simulink model "SEMINAR_DFIG_GSC_Controller"  (R2014a)
settings: Solver=ode45  StartTime=0.0  StopTime=10.0  RelTol=1e-3
libraries: powerlib_meascontrol x12, simulink x6
settings Model: Creator=user  LastModifiedBy=ninad gaikawad

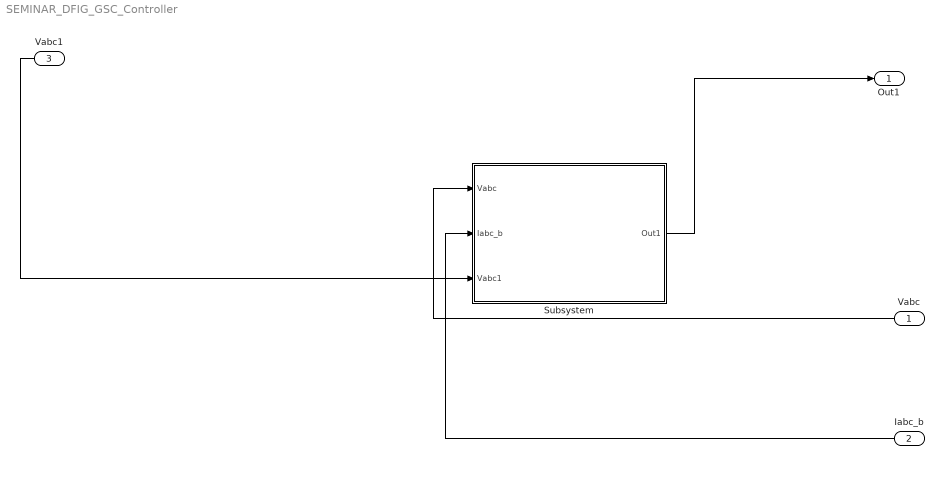
== system SEMINAR_DFIG_GSC_Controller ==
  Vabc : Inport
  Iabc_b : Inport  Port=2
  Vabc1 : Inport  Port=3
  Subsystem : Subsystem
  Out1 : Outport
  wires:
  Vabc/1 -> Subsystem/1(Vabc)
  Iabc_b/1 -> Subsystem/2(Iabc_b)
  Vabc1/1 -> Subsystem/3(Vabc1)
  Subsystem/1(Out1) -> Out1/1

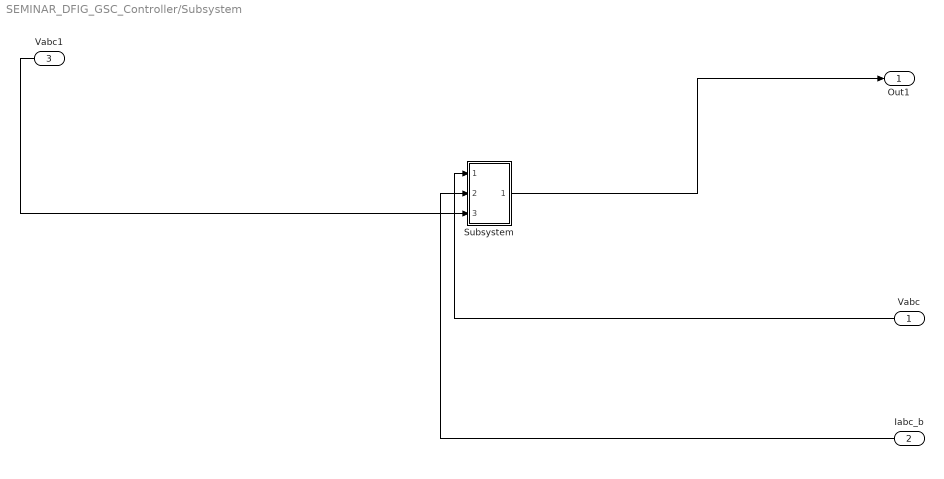
== system SEMINAR_DFIG_GSC_Controller/Subsystem ==
  Vabc : Inport
  Iabc_b : Inport  Port=2
  Vabc1 : Inport  Port=3
  Subsystem : Subsystem
  Out1 : Outport
  wires:
  Vabc/1 -> Subsystem/1(" Vabc_b")
  Iabc_b/1 -> Subsystem/2(Iabc_b)
  Vabc1/1 -> Subsystem/3
  Subsystem/1(pulses) -> Out1/1

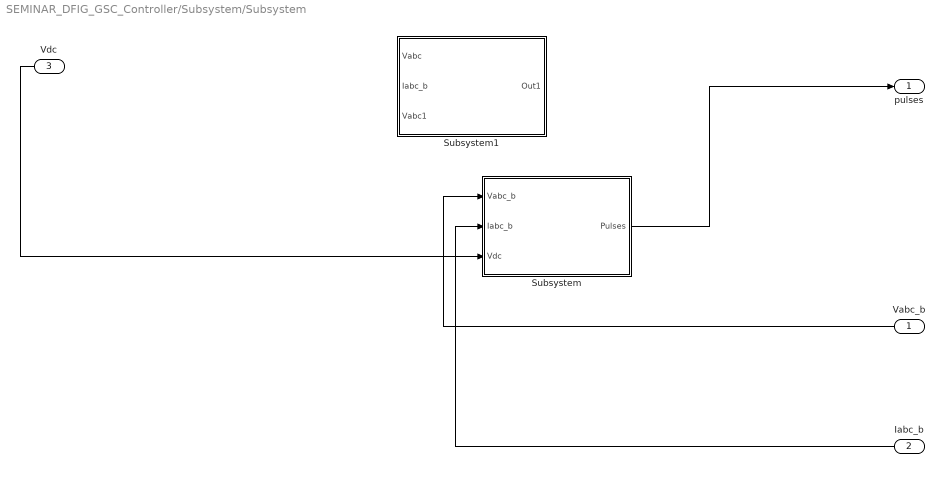
== system SEMINAR_DFIG_GSC_Controller/Subsystem/Subsystem ==
  " Vabc_b" : Inport
  Iabc_b : Inport  Port=2
  Vdc : Inport  Port=3 
  Subsystem : Subsystem
  Subsystem1 : Subsystem
  pulses : Outport
  wires:
  " Vabc_b"/1 -> Subsystem/1(Vabc_b)
  Iabc_b/1 -> Subsystem/2(Iabc_b)
  Vdc/1 -> Subsystem/3(Vdc)
  Subsystem/1(Pulses) -> pulses/1

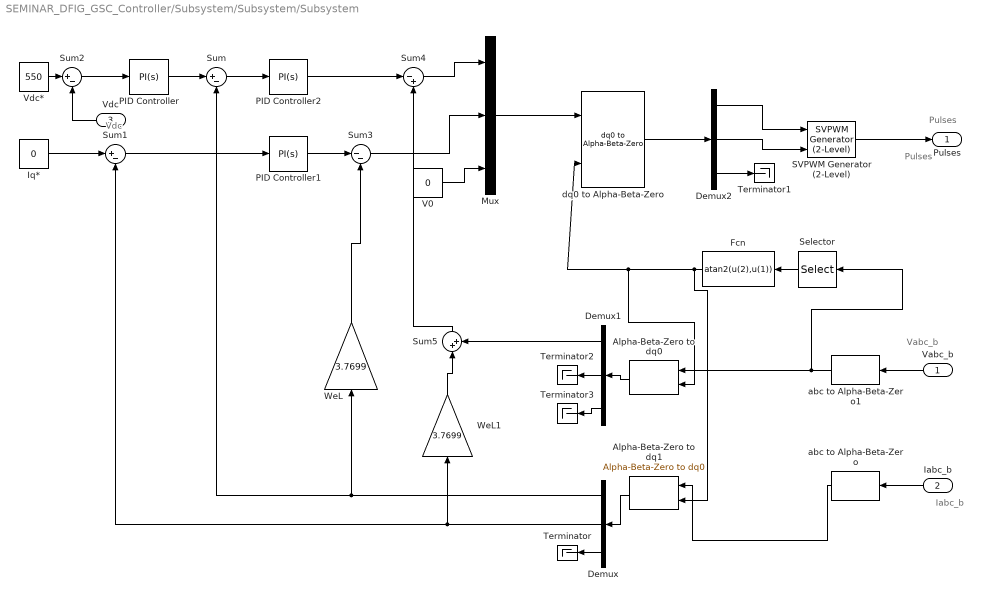
== system SEMINAR_DFIG_GSC_Controller/Subsystem/Subsystem/Subsystem ==
  note: Vdc
  note: Iabc_b
  note: Pulses
  note: Pulses
  note: Vabc_b
  Vabc_b : Inport
  Iabc_b : Inport  Port=2
  Vdc : Inport  Port=3
  Alpha-Beta-Zero to dq0 : powerlib_meascontrol/Transformations/Alpha-Beta-Zero to dq0  Alignment=Aligned with phase A axis
  Alpha-Beta-Zero to dq1 : powerlib_meascontrol/Transformations/Alpha-Beta-Zero to dq0  Alignment=Aligned with phase A axis
  Demux : Demux  Outputs=3
  Demux1 : Demux  Outputs=3
  Demux2 : Demux  Outputs=3
  Fcn : Fcn  Expr=atan2(u(2),u(1))
  Iq* : Constant  Value=0
  Mux : Mux  Inputs=3
  PID Controller : simulink/Continuous/PID Controller  Controller=PI  TimeDomain=Continuous-time  SampleTime=1  IntegratorMethod=Forward Euler  FilterMethod=Forward Euler  Form=Parallel  P=1  I=1  D=0  N=100  InitialConditionSource=internal  InitialConditionForIntegrator=0  InitialConditionForFilter=0  ExternalReset=none  LimitOutput=off  UpperSaturationLimit=inf  LowerSaturationLimit=-inf  LinearizeAsGain=on  AntiWindupMode=none  Kb=1  TrackingMode=off  Kt=1  PParamMin=[]  PParamMax=[]  IParamMin=[]  IParamMax=[]  DParamMin=[]  DParamMax=[]  NParamMin=[]  NParamMax=[]  KbParamMin=[]  KbParamMax=[]  KtParamMin=[]  KtParamMax=[]  POutMin=[]  POutMax=[]  IOutMin=[]  IOutMax=[]  DOutMin=[]  DOutMax=[]  NOutMin=[]  NOutMax=[]  KbOutMin=[]  KbOutMax=[]  KtOutMin=[]  KtOutMax=[]  IntegratorOutMin=[]  IntegratorOutMax=[]  FilterOutMin=[]  FilterOutMax=[]  SumOutMin=[]  SumOutMax=[]  SumI1OutMin=[]  SumI1OutMax=[]  SumI2OutMin=[]  SumI2OutMax=[]  SumI3OutMin=[]  SumI3OutMax=[]  SumDOutMin=[]  SumDOutMax=[]  SaturationOutMin=[]  SaturationOutMax=[]  IntegratorContinuousStateAttributes=''  IntegratorStateMustResolveToSignalObject=off  IntegratorRTWStateStorageClass=Auto  FilterContinuousStateAttributes=''  FilterStateMustResolveToSignalObject=off  FilterRTWStateStorageClass=Auto
  PID Controller1 : simulink/Continuous/PID Controller  Controller=PI  TimeDomain=Continuous-time  SampleTime=1  IntegratorMethod=Forward Euler  FilterMethod=Forward Euler  Form=Parallel  P=1  I=1  D=0  N=100  InitialConditionSource=internal  InitialConditionForIntegrator=0  InitialConditionForFilter=0  ExternalReset=none  LimitOutput=off  UpperSaturationLimit=inf  LowerSaturationLimit=-inf  LinearizeAsGain=on  AntiWindupMode=none  Kb=1  TrackingMode=off  Kt=1  PParamMin=[]  PParamMax=[]  IParamMin=[]  IParamMax=[]  DParamMin=[]  DParamMax=[]  NParamMin=[]  NParamMax=[]  KbParamMin=[]  KbParamMax=[]  KtParamMin=[]  KtParamMax=[]  POutMin=[]  POutMax=[]  IOutMin=[]  IOutMax=[]  DOutMin=[]  DOutMax=[]  NOutMin=[]  NOutMax=[]  KbOutMin=[]  KbOutMax=[]  KtOutMin=[]  KtOutMax=[]  IntegratorOutMin=[]  IntegratorOutMax=[]  FilterOutMin=[]  FilterOutMax=[]  SumOutMin=[]  SumOutMax=[]  SumI1OutMin=[]  SumI1OutMax=[]  SumI2OutMin=[]  SumI2OutMax=[]  SumI3OutMin=[]  SumI3OutMax=[]  SumDOutMin=[]  SumDOutMax=[]  SaturationOutMin=[]  SaturationOutMax=[]  IntegratorContinuousStateAttributes=''  IntegratorStateMustResolveToSignalObject=off  IntegratorRTWStateStorageClass=Auto  FilterContinuousStateAttributes=''  FilterStateMustResolveToSignalObject=off  FilterRTWStateStorageClass=Auto
  PID Controller2 : simulink/Continuous/PID Controller  Controller=PI  TimeDomain=Continuous-time  SampleTime=1  IntegratorMethod=Forward Euler  FilterMethod=Forward Euler  Form=Parallel  P=1  I=1  D=0  N=100  InitialConditionSource=internal  InitialConditionForIntegrator=0  InitialConditionForFilter=0  ExternalReset=none  LimitOutput=off  UpperSaturationLimit=inf  LowerSaturationLimit=-inf  LinearizeAsGain=on  AntiWindupMode=none  Kb=1  TrackingMode=off  Kt=1  PParamMin=[]  PParamMax=[]  IParamMin=[]  IParamMax=[]  DParamMin=[]  DParamMax=[]  NParamMin=[]  NParamMax=[]  KbParamMin=[]  KbParamMax=[]  KtParamMin=[]  KtParamMax=[]  POutMin=[]  POutMax=[]  IOutMin=[]  IOutMax=[]  DOutMin=[]  DOutMax=[]  NOutMin=[]  NOutMax=[]  KbOutMin=[]  KbOutMax=[]  KtOutMin=[]  KtOutMax=[]  IntegratorOutMin=[]  IntegratorOutMax=[]  FilterOutMin=[]  FilterOutMax=[]  SumOutMin=[]  SumOutMax=[]  SumI1OutMin=[]  SumI1OutMax=[]  SumI2OutMin=[]  SumI2OutMax=[]  SumI3OutMin=[]  SumI3OutMax=[]  SumDOutMin=[]  SumDOutMax=[]  SaturationOutMin=[]  SaturationOutMax=[]  IntegratorContinuousStateAttributes=''  IntegratorStateMustResolveToSignalObject=off  IntegratorRTWStateStorageClass=Auto  FilterContinuousStateAttributes=''  FilterStateMustResolveToSignalObject=off  FilterRTWStateStorageClass=Auto
  SVPWM Generator (2-Level) : powerlib_meascontrol/Pulse & Signal Generators/SVPWM Generator (2-Level)  InputType=alpha-beta components  SwitchingPattern=Pattern #1  Fc=27*50  ParUref=[0.8 -30 50]  Ts=0
  Selector : Selector  InputPortWidth=3  Indices=[1 2]
  Sum : Sum  Inputs=|+-
  Sum1 : Sum  Inputs=|+-
  Sum2 : Sum  Inputs=|+-
  Sum3 : Sum  Inputs=|--
  Sum4 : Sum  Inputs=|-+
  Sum5 : Sum  Inputs=|++
  Terminator{,1..3} (4 alike) : Terminator
  V0 : Constant  Value=0
  Vdc* : Constant  Value=550
  WeL : Gain  Gain=3.7699
  WeL1 : Gain  Gain=3.7699
  abc to Alpha-Beta-Zero : powerlib_meascontrol/Transformations/abc to Alpha-Beta-Zero
  abc to Alpha-Beta-Zero1 : powerlib_meascontrol/Transformations/abc to Alpha-Beta-Zero
  dq0 to Alpha-Beta-Zero : powerlib_meascontrol/Transformations/dq0 to Alpha-Beta-Zero  Alignment=90 degrees behind phase A axis
  Pulses : Outport
  wires:
  Demux1/3 -> Terminator3/1
  Demux/3 -> Terminator/1
  Alpha-Beta-Zero to dq1/1 -> Demux/1
  Fcn/1 -> Alpha-Beta-Zero to dq1/2, dq0 to Alpha-Beta-Zero/2, Alpha-Beta-Zero to dq0/2
  abc to Alpha-Beta-Zero1/1 -> Selector/1, Alpha-Beta-Zero to dq0/1
  abc to Alpha-Beta-Zero/1 -> Alpha-Beta-Zero to dq1/1
  Alpha-Beta-Zero to dq0/1 -> Demux1/1
  Vabc_b/1 -> abc to Alpha-Beta-Zero1/1
  Demux1/2 -> Terminator2/1
  Iabc_b/1 -> abc to Alpha-Beta-Zero/1
  Selector/1 -> Fcn/1
  Demux2/3 -> Terminator1/1
  Demux2/2 -> SVPWM Generator (2-Level)/2
  Demux2/1 -> SVPWM Generator (2-Level)/1
  dq0 to Alpha-Beta-Zero/1 -> Demux2/1
  SVPWM Generator (2-Level)/1 -> Pulses/1
  Mux/1 -> dq0 to Alpha-Beta-Zero/1
  Sum4/1 -> Mux/1
  PID Controller1/1 -> Sum3/1
  Demux/1 -> WeL/1, Sum/2
  Demux1/1 -> Sum5/2
  PID Controller2/1 -> Sum4/1
  Vdc/1 -> Sum2/2
  Demux/2 -> WeL1/1, Sum1/2
  Sum1/1 -> PID Controller1/1
  Sum5/1 -> Sum4/2
  Sum3/1 -> Mux/2
  WeL1/1 -> Sum5/1
  PID Controller/1 -> Sum/1
  Iq*/1 -> Sum1/1
  WeL/1 -> Sum3/2
  Sum2/1 -> PID Controller/1
  Vdc*/1 -> Sum2/1
  V0/1 -> Mux/3
  Sum/1 -> PID Controller2/1

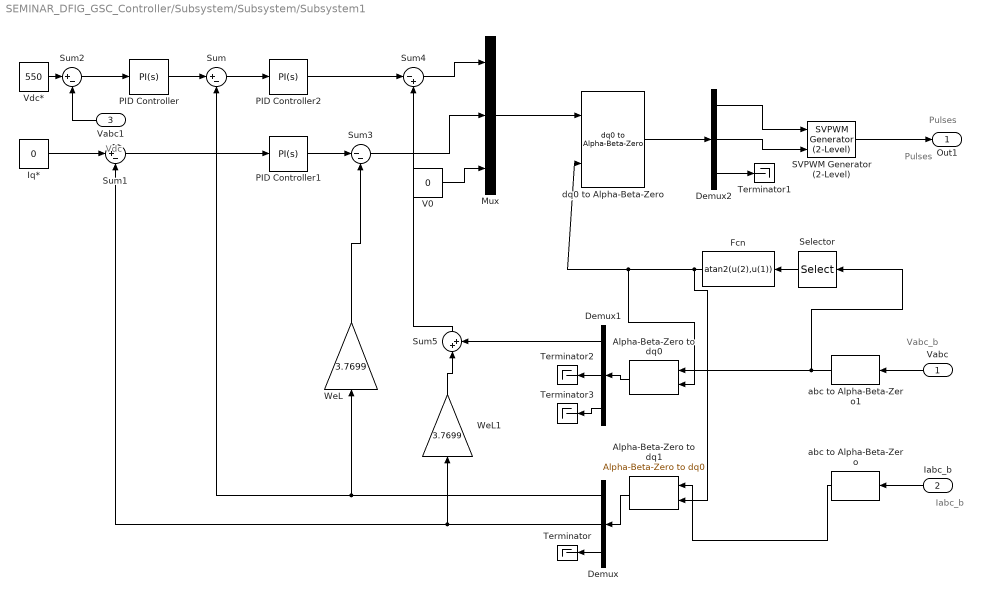
== system SEMINAR_DFIG_GSC_Controller/Subsystem/Subsystem/Subsystem1 ==
  note: Vdc
  note: Iabc_b
  note: Pulses
  note: Pulses
  note: Vabc_b
  Vabc : Inport
  Iabc_b : Inport  Port=2
  Vabc1 : Inport  Port=3
  Alpha-Beta-Zero to dq0 : powerlib_meascontrol/Transformations/Alpha-Beta-Zero to dq0  Alignment=Aligned with phase A axis
  Alpha-Beta-Zero to dq1 : powerlib_meascontrol/Transformations/Alpha-Beta-Zero to dq0  Alignment=Aligned with phase A axis
  Demux : Demux  Outputs=3
  Demux1 : Demux  Outputs=3
  Demux2 : Demux  Outputs=3
  Fcn : Fcn  Expr=atan2(u(2),u(1))
  Iq* : Constant  Value=0
  Mux : Mux  Inputs=3
  PID Controller : simulink/Continuous/PID Controller  Controller=PI  TimeDomain=Continuous-time  SampleTime=1  IntegratorMethod=Forward Euler  FilterMethod=Forward Euler  Form=Parallel  P=1  I=1  D=0  N=100  InitialConditionSource=internal  InitialConditionForIntegrator=0  InitialConditionForFilter=0  ExternalReset=none  LimitOutput=off  UpperSaturationLimit=inf  LowerSaturationLimit=-inf  LinearizeAsGain=on  AntiWindupMode=none  Kb=1  TrackingMode=off  Kt=1  PParamMin=[]  PParamMax=[]  IParamMin=[]  IParamMax=[]  DParamMin=[]  DParamMax=[]  NParamMin=[]  NParamMax=[]  KbParamMin=[]  KbParamMax=[]  KtParamMin=[]  KtParamMax=[]  POutMin=[]  POutMax=[]  IOutMin=[]  IOutMax=[]  DOutMin=[]  DOutMax=[]  NOutMin=[]  NOutMax=[]  KbOutMin=[]  KbOutMax=[]  KtOutMin=[]  KtOutMax=[]  IntegratorOutMin=[]  IntegratorOutMax=[]  FilterOutMin=[]  FilterOutMax=[]  SumOutMin=[]  SumOutMax=[]  SumI1OutMin=[]  SumI1OutMax=[]  SumI2OutMin=[]  SumI2OutMax=[]  SumI3OutMin=[]  SumI3OutMax=[]  SumDOutMin=[]  SumDOutMax=[]  SaturationOutMin=[]  SaturationOutMax=[]  IntegratorContinuousStateAttributes=''  IntegratorStateMustResolveToSignalObject=off  IntegratorRTWStateStorageClass=Auto  FilterContinuousStateAttributes=''  FilterStateMustResolveToSignalObject=off  FilterRTWStateStorageClass=Auto
  PID Controller1 : simulink/Continuous/PID Controller  Controller=PI  TimeDomain=Continuous-time  SampleTime=1  IntegratorMethod=Forward Euler  FilterMethod=Forward Euler  Form=Parallel  P=1  I=1  D=0  N=100  InitialConditionSource=internal  InitialConditionForIntegrator=0  InitialConditionForFilter=0  ExternalReset=none  LimitOutput=off  UpperSaturationLimit=inf  LowerSaturationLimit=-inf  LinearizeAsGain=on  AntiWindupMode=none  Kb=1  TrackingMode=off  Kt=1  PParamMin=[]  PParamMax=[]  IParamMin=[]  IParamMax=[]  DParamMin=[]  DParamMax=[]  NParamMin=[]  NParamMax=[]  KbParamMin=[]  KbParamMax=[]  KtParamMin=[]  KtParamMax=[]  POutMin=[]  POutMax=[]  IOutMin=[]  IOutMax=[]  DOutMin=[]  DOutMax=[]  NOutMin=[]  NOutMax=[]  KbOutMin=[]  KbOutMax=[]  KtOutMin=[]  KtOutMax=[]  IntegratorOutMin=[]  IntegratorOutMax=[]  FilterOutMin=[]  FilterOutMax=[]  SumOutMin=[]  SumOutMax=[]  SumI1OutMin=[]  SumI1OutMax=[]  SumI2OutMin=[]  SumI2OutMax=[]  SumI3OutMin=[]  SumI3OutMax=[]  SumDOutMin=[]  SumDOutMax=[]  SaturationOutMin=[]  SaturationOutMax=[]  IntegratorContinuousStateAttributes=''  IntegratorStateMustResolveToSignalObject=off  IntegratorRTWStateStorageClass=Auto  FilterContinuousStateAttributes=''  FilterStateMustResolveToSignalObject=off  FilterRTWStateStorageClass=Auto
  PID Controller2 : simulink/Continuous/PID Controller  Controller=PI  TimeDomain=Continuous-time  SampleTime=1  IntegratorMethod=Forward Euler  FilterMethod=Forward Euler  Form=Parallel  P=1  I=1  D=0  N=100  InitialConditionSource=internal  InitialConditionForIntegrator=0  InitialConditionForFilter=0  ExternalReset=none  LimitOutput=off  UpperSaturationLimit=inf  LowerSaturationLimit=-inf  LinearizeAsGain=on  AntiWindupMode=none  Kb=1  TrackingMode=off  Kt=1  PParamMin=[]  PParamMax=[]  IParamMin=[]  IParamMax=[]  DParamMin=[]  DParamMax=[]  NParamMin=[]  NParamMax=[]  KbParamMin=[]  KbParamMax=[]  KtParamMin=[]  KtParamMax=[]  POutMin=[]  POutMax=[]  IOutMin=[]  IOutMax=[]  DOutMin=[]  DOutMax=[]  NOutMin=[]  NOutMax=[]  KbOutMin=[]  KbOutMax=[]  KtOutMin=[]  KtOutMax=[]  IntegratorOutMin=[]  IntegratorOutMax=[]  FilterOutMin=[]  FilterOutMax=[]  SumOutMin=[]  SumOutMax=[]  SumI1OutMin=[]  SumI1OutMax=[]  SumI2OutMin=[]  SumI2OutMax=[]  SumI3OutMin=[]  SumI3OutMax=[]  SumDOutMin=[]  SumDOutMax=[]  SaturationOutMin=[]  SaturationOutMax=[]  IntegratorContinuousStateAttributes=''  IntegratorStateMustResolveToSignalObject=off  IntegratorRTWStateStorageClass=Auto  FilterContinuousStateAttributes=''  FilterStateMustResolveToSignalObject=off  FilterRTWStateStorageClass=Auto
  SVPWM Generator (2-Level) : powerlib_meascontrol/Pulse & Signal Generators/SVPWM Generator (2-Level)  InputType=alpha-beta components  SwitchingPattern=Pattern #1  Fc=27*50  ParUref=[0.8 -30 50]  Ts=0
  Selector : Selector  InputPortWidth=3  Indices=[1 2]
  Sum : Sum  Inputs=|+-
  Sum1 : Sum  Inputs=|+-
  Sum2 : Sum  Inputs=|+-
  Sum3 : Sum  Inputs=|--
  Sum4 : Sum  Inputs=|-+
  Sum5 : Sum  Inputs=|++
  Terminator{,1..3} (4 alike) : Terminator
  V0 : Constant  Value=0
  Vdc* : Constant  Value=550
  WeL : Gain  Gain=3.7699
  WeL1 : Gain  Gain=3.7699
  abc to Alpha-Beta-Zero : powerlib_meascontrol/Transformations/abc to Alpha-Beta-Zero
  abc to Alpha-Beta-Zero1 : powerlib_meascontrol/Transformations/abc to Alpha-Beta-Zero
  dq0 to Alpha-Beta-Zero : powerlib_meascontrol/Transformations/dq0 to Alpha-Beta-Zero  Alignment=90 degrees behind phase A axis
  Out1 : Outport
  wires:
  Demux1/3 -> Terminator3/1
  Demux/3 -> Terminator/1
  Alpha-Beta-Zero to dq1/1 -> Demux/1
  Fcn/1 -> Alpha-Beta-Zero to dq1/2, dq0 to Alpha-Beta-Zero/2, Alpha-Beta-Zero to dq0/2
  abc to Alpha-Beta-Zero1/1 -> Selector/1, Alpha-Beta-Zero to dq0/1
  abc to Alpha-Beta-Zero/1 -> Alpha-Beta-Zero to dq1/1
  Alpha-Beta-Zero to dq0/1 -> Demux1/1
  Vabc/1 -> abc to Alpha-Beta-Zero1/1
  Demux1/2 -> Terminator2/1
  Iabc_b/1 -> abc to Alpha-Beta-Zero/1
  Selector/1 -> Fcn/1
  Demux2/3 -> Terminator1/1
  Demux2/2 -> SVPWM Generator (2-Level)/2
  Demux2/1 -> SVPWM Generator (2-Level)/1
  dq0 to Alpha-Beta-Zero/1 -> Demux2/1
  SVPWM Generator (2-Level)/1 -> Out1/1
  Mux/1 -> dq0 to Alpha-Beta-Zero/1
  Sum4/1 -> Mux/1
  PID Controller1/1 -> Sum3/1
  Demux/1 -> WeL/1, Sum/2
  Demux1/1 -> Sum5/2
  PID Controller2/1 -> Sum4/1
  Vabc1/1 -> Sum2/2
  Demux/2 -> WeL1/1, Sum1/2
  Sum1/1 -> PID Controller1/1
  Sum5/1 -> Sum4/2
  Sum3/1 -> Mux/2
  WeL1/1 -> Sum5/1
  PID Controller/1 -> Sum/1
  Iq*/1 -> Sum1/1
  WeL/1 -> Sum3/2
  Sum2/1 -> PID Controller/1
  Vdc*/1 -> Sum2/1
  V0/1 -> Mux/3
  Sum/1 -> PID Controller2/1
